simulink model "Mophong_Daodong_1phan4"  (R2021b)
settings: Solver=VariableStepAuto  StartTime=0.0  StopTime=50  RelTol=1e-3
undefined symbols (not defined in the file): c, k, m, q, w
settings Model: Creator=jackl  LastModifiedBy=jackl

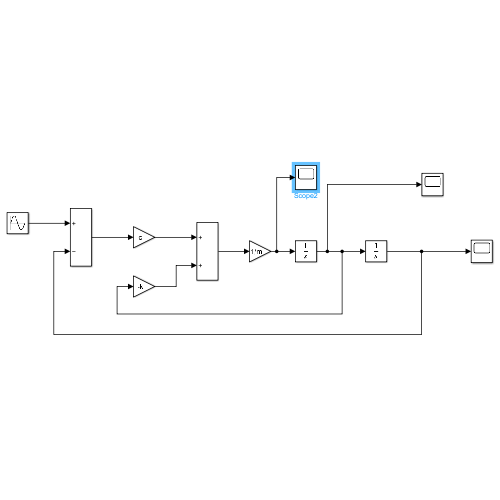
[thumbnail: Simulink's stored preview of the top-level diagram]
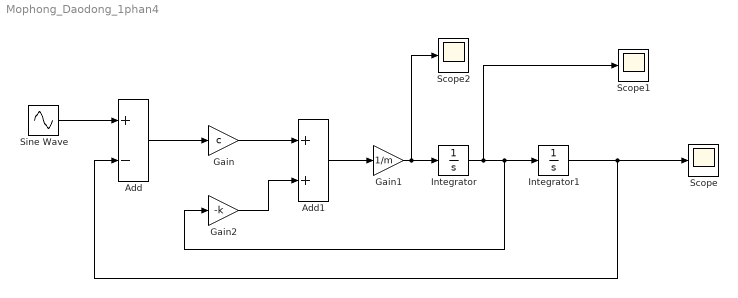
== system Mophong_Daodong_1phan4 ==
  Add : Sum  Inputs=+-
  Add1 : Sum
  Gain : Gain  Gain=c
  Gain1 : Gain  Gain=1/m
  Gain2 : Gain  Gain=-k
  Integrator : Integrator
  Integrator1 : Integrator
  Scope : Scope
  Scope1 : Scope
  Scope2 : Scope
  Sine Wave : Sin  Amplitude=q  Frequency=w  SampleTime=0
  wires:
  Integrator/1 -> Scope1/1, Gain2/1, Integrator1/1
  Integrator1/1 -> Scope/1, Add/2
  Add1/1 -> Gain1/1
  Gain1/1 -> Scope2/1, Integrator/1
  Gain/1 -> Add1/1
  Add/1 -> Gain/1
  Sine Wave/1 -> Add/1
  Gain2/1 -> Add1/2
